simulink model "DC motor speed control"  (R2021a)
settings: Solver=VariableStepAuto  StartTime=0.0  StopTime=5  RelTol=1e-3
values from neighbouring files (symbols this model uses):
  c1 = 18.2645    [control of EV3 robot using speed voltage relationship.m]
  c2 = 0.9945    [control of EV3 robot using speed voltage relationship.m]
settings Model: Creator=hritw  LastModifiedBy=hritw

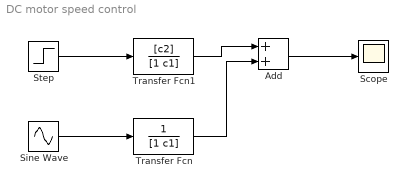
== system DC motor speed control ==
  Add : Sum
  Scope : Scope
  Sine Wave : Sin  Amplitude=-0.2  Frequency=4*pi*(10^6)  Phase=-pi/2  SampleTime=0
  Step : Step  After=5  SampleTime=0
  Transfer Fcn : TransferFcn  Denominator=[1 c1]
  Transfer Fcn1 : TransferFcn  Numerator=[c2]  Denominator=[1 c1]
  wires:
  Step/1 -> Transfer Fcn1/1
  Add/1 -> Scope/1
  Transfer Fcn1/1 -> Add/1
  Transfer Fcn/1 -> Add/2
  Sine Wave/1 -> Transfer Fcn/1
